simulink model "Get_RE_RhythmCalc_Sig2Mbed_plotdAV"  (R2013a)
settings: Solver=FixedStepDiscrete  StartTime=0.0  StopTime=60  RelTol=1e-3
undefined symbols (not defined in the file): ts
libraries: arduino_io_lib x12, simulink x3
settings Model: Creator=cell  LastModifiedBy=cell
settings OptimizationCC: OptimizeModelRefInitCode=on  LifeSpan=1
settings DebuggingCC: StrictBusMsg=Warning
settings HardwareCC: ProdBitPerInt=16  ProdBitPerPointer=8  ProdIntDivRoundTo=Zero  ProdEndianess=LittleEndian  ProdWordSize=8  ProdHWDeviceType=Atmel->AVR
settings RTWCC: SystemTargetFile=realtime.tlc  GenerateMakefile=off  TemplateMakefile=realtime.tmf  Description=Run on Target Hardware  RTWVerbose=off  ProcessScript=realtime_make_rtw_hook
settings CodeAppCC: IgnoreCustomStorageClasses=off
settings STFCustomTargetCC: TargetLibSuffix=.a  GenerateSampleERTMain=on  CombineOutputUpdateFcns=on  ERTCustomFileBanners=on  SupportContinuousTime=off  SupportNonInlinedSFcns=off  MATLABClassNameForMDSCustomization=Simulink.SoftwareTarget.ERTCustomization  SystemTargetFile=realtime.tlc
settings ERTTargetCC: ParMdlRefBuildCompliant=off  CompOptLevelCompliant=off  ConcurrentExecutionCompliant=off  ERTFirstTimeCompliant=off  ModelStepFunctionPrototypeControlCompliant=off  CPPClassGenCompliant=off  ERTCustomFileTemplate=realtime_file_process.tlc

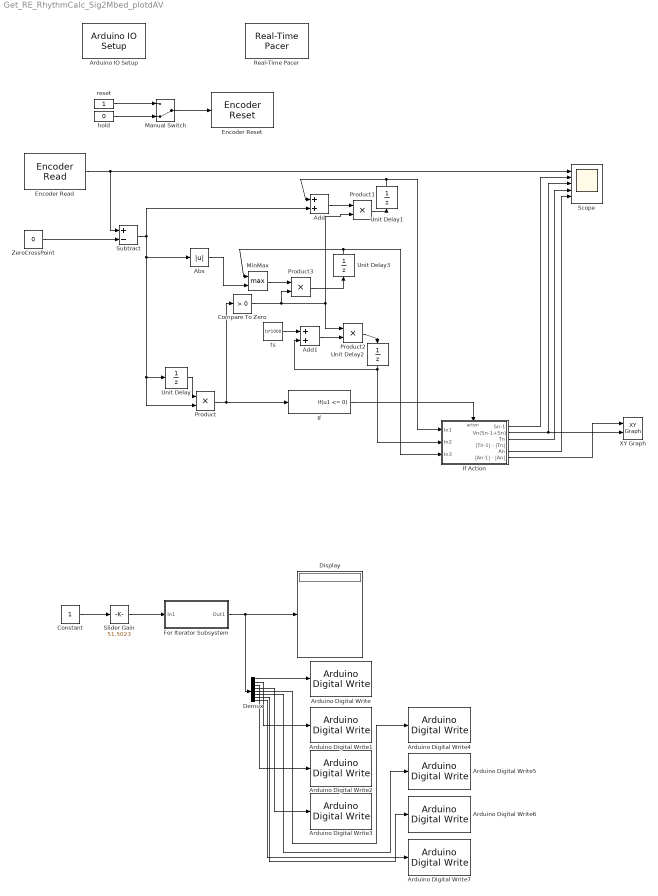
== system Get_RE_RhythmCalc_Sig2Mbed_plotdAV ==
  Abs : Abs
  Add : Sum
  Add1 : Sum
  Arduino Digital Write : arduino_io_lib/Arduino Digital Write  arduinoVar=Existing workspace arduino variable #1  arduinoPin=6  T=ts
  Arduino Digital Write1 : arduino_io_lib/Arduino Digital Write  arduinoVar=Existing workspace arduino variable #1  arduinoPin=7  T=ts
  Arduino Digital Write2 : arduino_io_lib/Arduino Digital Write  arduinoVar=Existing workspace arduino variable #1  arduinoPin=8  T=ts
  Arduino Digital Write3 : arduino_io_lib/Arduino Digital Write  arduinoVar=Existing workspace arduino variable #1  arduinoPin=9  T=ts
  Arduino Digital Write4 : arduino_io_lib/Arduino Digital Write  arduinoVar=Existing workspace arduino variable #1  arduinoPin=10  T=ts
  Arduino Digital Write5 : arduino_io_lib/Arduino Digital Write  arduinoVar=Existing workspace arduino variable #1  arduinoPin=11  T=ts
  Arduino Digital Write6 : arduino_io_lib/Arduino Digital Write  arduinoVar=Existing workspace arduino variable #1  arduinoPin=12  T=ts
  Arduino Digital Write7 : arduino_io_lib/Arduino Digital Write  arduinoVar=Existing workspace arduino variable #1  arduinoPin=13  T=ts
  Arduino IO Setup : arduino_io_lib/Arduino IO Setup  Priority=3  arduinoVar=Existing workspace arduino variable #1  workspaceVarName=a  comPort=DEMO
  Compare To Zero : simulink/Logic and Bit Operations/Compare To Zero  relop=>  OutDataTypeStr=boolean
  Constant : Constant
  Demux : Demux  Outputs=8
  Display : Display
  Encoder Read : arduino_io_lib/Encoder Read  arduinoVar=Existing workspace arduino variable #1  encNum=1  pinA=2  pinB=3  DbDl=0  T=ts
  Encoder Reset : arduino_io_lib/Encoder Reset  arduinoVar=Existing workspace arduino variable #1  encNum=1  T=ts
  For Iterator Subsystem : Subsystem  TreatAsAtomicUnit=on  mask{bits=8}
      mask prompts: bits "ビット数"
      mask Display: disp('Integer To Bit\nConvertor')
  If : If  IfExpression=u1 <= 0  ShowElse=off
  "If Action " : Subsystem  TreatAsAtomicUnit=on
  Manual Switch : ManualSwitch  CurrentSetting=0
  MinMax : MinMax  Function=max  Inputs=2  OutDataTypeStr=double
      settings: LockScale=on
  Product{,1..3} (4 alike) : Product
  Real-Time Pacer : arduino_io_lib/Real-Time Pacer  simTimePerRealTime=1
  Scope : Scope  NumInputPorts=5
      settings: TimeRange=10  YMin=-300~-1750~-1750~0~0  YMax=250~1750~1500~250~275
  Slider Gain : simulink/Math Operations/Slider Gain  low=0  gain=51.5023  high=254
  Subtract : Sum  Inputs=+-
  Unit Delay{,1..3} (4 alike) : UnitDelay  SampleTime=-1
  XY Graph : simulink/Sinks/XY Graph  xmin=0  xmax=500  ymin=0  ymax=50000  st=-1
  ZeroCrossPoint : Constant  Value=0
  hold : Constant  Value=0
  reset : Constant
  ts : Constant  Value=ts*1000
  wires:
  reset/1 -> Manual Switch/1
  hold/1 -> Manual Switch/2
  Manual Switch/1 -> Encoder Reset/1
  Encoder Read/1 -> Subtract/1, Scope/1
  For Iterator Subsystem/1(Out1) -> Demux/1, Display/1
  Demux/1 -> Arduino Digital Write/1
  Demux/2 -> Arduino Digital Write1/1
  Demux/3 -> Arduino Digital Write2/1
  Demux/4 -> Arduino Digital Write3/1
  Demux/5 -> Arduino Digital Write4/1
  Demux/6 -> Arduino Digital Write5/1
  Demux/7 -> Arduino Digital Write6/1
  Demux/8 -> Arduino Digital Write7/1
  Unit Delay/1 -> Product/1
  ZeroCrossPoint/1 -> Subtract/2
  If/1 -> "If Action "/Action
  Product/1 -> If/1, Compare To Zero/1
  Subtract/1 -> Product/2, Unit Delay/1, Abs/1, Add/2
  Product1/1 -> Unit Delay1/1
  Constant/1 -> Slider Gain/1
  Slider Gain/1 -> For Iterator Subsystem/1(In1)
  "If Action "/1(Sn-1) -> Scope/2
  Compare To Zero/1 -> Product3/2, Product1/2, Product2/1
  Unit Delay2/1 -> Add1/2, "If Action "/2(In2)
  Add1/1 -> Product2/2
  Product2/1 -> Unit Delay2/1
  ts/1 -> Add1/1
  Unit Delay1/1 -> Add/1, "If Action "/1(In1)
  Add/1 -> Product1/1
  "If Action "/3(Tn) -> Scope/4
  Abs/1 -> MinMax/2
  "If Action "/5(An) -> Scope/5
  Unit Delay3/1 -> MinMax/1, "If Action "/3(In3)
  MinMax/1 -> Product3/1
  Product3/1 -> Unit Delay3/1
  "If Action "/2(Vn(Sn-1+Sn)) -> XY Graph/2, Scope/3
  "If Action "/6(|An-1| - |An|) -> XY Graph/1

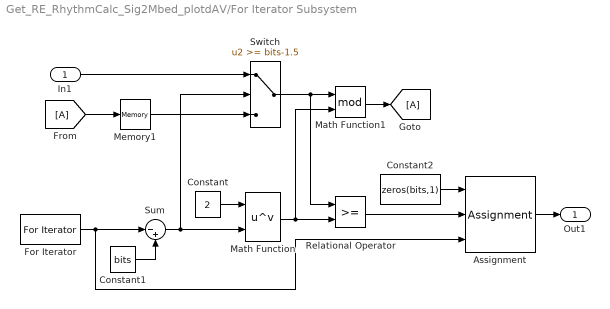
== system Get_RE_RhythmCalc_Sig2Mbed_plotdAV/For Iterator Subsystem ==
  In1 : Inport
  Assignment : Assignment  IndexOptions=Index vector (port)  Indices=1  OutputSizes=[1 1]
  Constant : Constant  Value=2
  Constant1 : Constant  Value=bits
  Constant2 : Constant  Value=zeros(bits,1)  VectorParams1D=off
  For Iterator : ForIterator  IterationLimit=bits
  Math Function : Math  Operator=pow  SaturateOnIntegerOverflow=on
  Math Function1 : Math  Operator=mod  SaturateOnIntegerOverflow=on
  Memory1 : Memory  InheritSampleTime=on
  Relational Operator : RelationalOperator  OutDataTypeStr=float('double')
  Sum : Sum  Inputs=|-+
  Switch : Switch  Threshold=bits-1.5
  Out1 : Outport
  wires:
  For Iterator/1 -> Sum/1, Assignment/3
  Constant/1 -> Math Function/1
  Sum/1 -> Math Function/2, Switch/2
  Constant1/1 -> Sum/2
  Math Function/1 -> Math Function1/2, Relational Operator/2
  Switch/1 -> Math Function1/1, Relational Operator/1
  In1/1 -> Switch/1
  Memory1/1 -> Switch/3
  Assignment/1 -> Out1/1
  Constant2/1 -> Assignment/1
  Relational Operator/1 -> Assignment/2
  [A] -> Memory1/1
  Math Function1/1 -> [A]

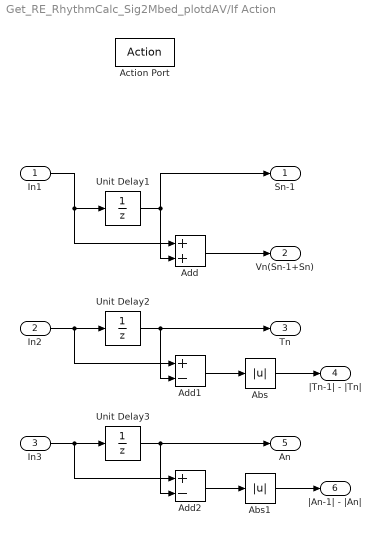
== system Get_RE_RhythmCalc_Sig2Mbed_plotdAV/If Action  ==
  In1 : Inport
  In2 : Inport  Port=2
  In3 : Inport  Port=3
  Action Port : ActionPort  ActionType=then
  Abs : Abs
  Abs1 : Abs
  Add : Sum
  Add1 : Sum  Inputs=+-
  Add2 : Sum  Inputs=+-
  Unit Delay1 : UnitDelay  SampleTime=-1
  Unit Delay2 : UnitDelay  SampleTime=-1
  Unit Delay3 : UnitDelay  SampleTime=-1
  Sn-1 : Outport
  Vn(Sn-1+Sn) : Outport  Port=2
  Tn : Outport  Port=3
  |Tn-1| - |Tn| : Outport  Port=4
  An : Outport  Port=5
  |An-1| - |An| : Outport  Port=6
  wires:
  Unit Delay1/1 -> Sn-1/1, Add/2
  In1/1 -> Add/1, Unit Delay1/1
  Add/1 -> Vn(Sn-1+Sn)/1
  Unit Delay2/1 -> Add1/2, Tn/1
  In2/1 -> Add1/1, Unit Delay2/1
  Add1/1 -> Abs/1
  Abs/1 -> |Tn-1| - |Tn|/1
  Unit Delay3/1 -> An/1, Add2/2
  In3/1 -> Unit Delay3/1, Add2/1
  Add2/1 -> Abs1/1
  Abs1/1 -> |An-1| - |An|/1
